simulink model "attitude_drone"  (R2022b)
settings: Solver=VariableStepAuto  StartTime=0.0  StopTime=10.0  RelTol=1e-3
settings Model: Creator=efloresm  LastModifiedBy=efloresm

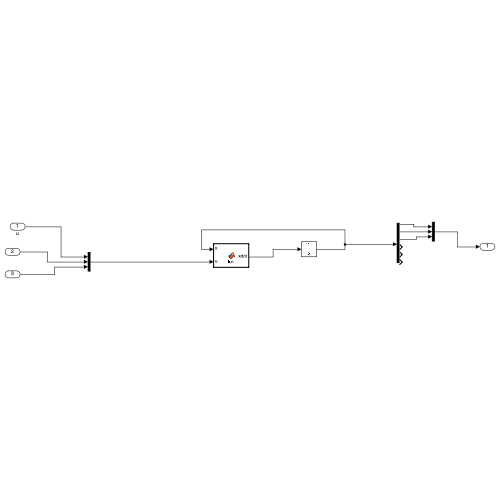
[thumbnail: Simulink's stored preview of the top-level diagram]
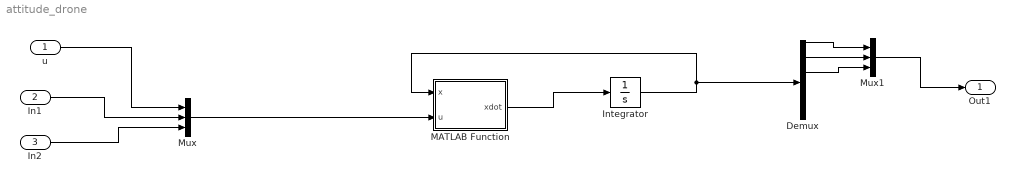
== system attitude_drone ==
  u : Inport
  In1 : Inport  Port=2
  In2 : Inport  Port=3
  Demux : Demux  Outputs=6
  Integrator : Integrator
  MATLAB Function : MATLAB Function  TreatAsAtomicUnit=on
  Mux : Mux  Inputs=3
  Mux1 : Mux  Inputs=3
  Out1 : Outport
  wires:
  MATLAB Function/1(xdot) -> Integrator/1
  Integrator/1 -> Demux/1, MATLAB Function/1(x)
  Mux/1 -> MATLAB Function/2(u)
  u/1 -> Mux/1
  In1/1 -> Mux/2
  In2/1 -> Mux/3
  Demux/1 -> Mux1/1
  Demux/2 -> Mux1/2
  Demux/3 -> Mux1/3
  Mux1/1 -> Out1/1

== matlab function attitude_drone/MATLAB Function ==
  data: x input; u input; xdot output
function xdot = fcn(x,u)

xdot = zeros(6,1);
% Extract state variables from state vector
roll    = x(1);
pitch   = x(2);
yaw     = x(3);
omega_x = x(4);
omega_y = x(5);
omega_z = x(6);

% Inertia moments
Jx = 0.1;
Jy = 0.1;
Jz = 0.2;



%%%%%%%%%%%%%%%%%%%%%%%%%%%%%

tau_roll    = u(1);
tau_pitch   = u(2);
tau_yaw     = u(3);

%%%%%%%%%%%%%%%%%%%%%%%%%%%%%%

roll_dot    = omega_x + sin(roll)*tan(pitch)*omega_y + cos(roll)*tan(pitch)*omega_z;
pitch_dot   =         +            cos(roll)*omega_y -            sin(roll)*omega_z;
yaw_dot     =         + sin(roll)/cos(pitch)*omega_y + cos(roll)/cos(pitch)*omega_z;


omega_x_dot = (Jy - Jz)/Jx*omega_y*omega_z + tau_roll/Jx;
omega_y_dot = (Jx - Jz)/Jy*omega_x*omega_z + tau_pitch/Jy;
omega_z_dot = (Jx - Jy)/Jz*omega_x*omega_y + tau_yaw/Jz;

xdot(1) = roll_dot;
xdot(2) = pitch_dot;
xdot(3) = yaw_dot;
xdot(4) = omega_x_dot;
xdot(5) = omega_y_dot;
xdot(6) = omega_z_dot;
